simulink model "Concentrationlambdasum"  (R2020a)
settings: Solver=VariableStepAuto  StartTime=0.0  StopTime=10.0  RelTol=1e-3
undefined symbols (not defined in the file): beta1, beta2, beta3, beta4, beta5, beta6, lambda1, lambda2, lambda3, lambda4, lambda5, lambda6, mean_prompt_neutron_gen_t
settings Model: Creator=marce  LastModifiedBy=tkdmc

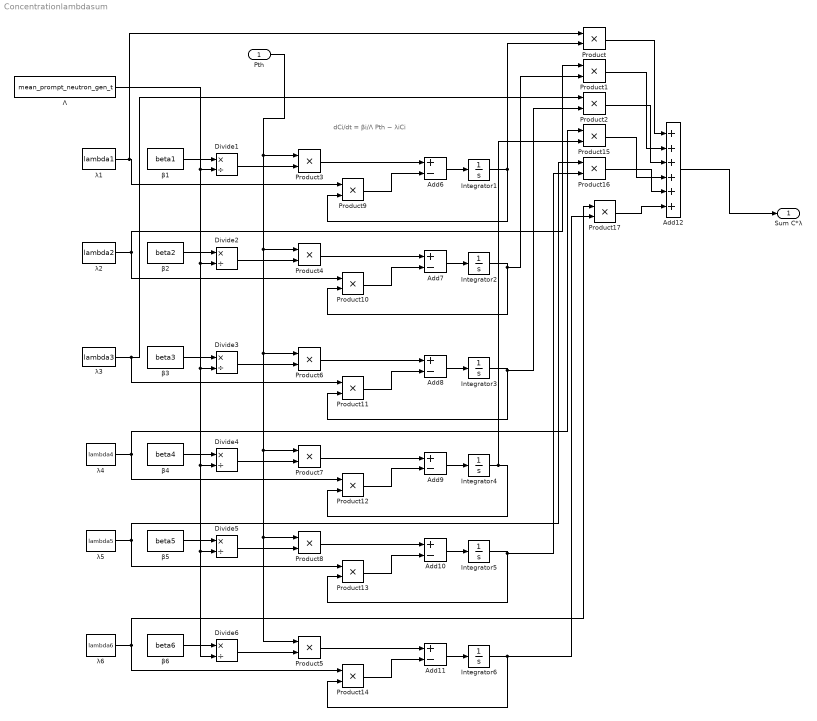
== system Concentrationlambdasum ==
  note: dCi/dt = βi/Λ Pth − λiCi
  Pth : Inport
  Add{6..11} (6 alike) : Sum  Inputs=+-
  Add12 : Sum  Inputs=++++++
  Divide{1..6} (6 alike) : Product  Inputs=*/
  Integrator{1..6} (6 alike) : Integrator
  Product{,1..17} (18 alike) : Product
  "Λ " : Constant  Value=mean_prompt_neutron_gen_t
  β1 : Constant  Value=beta1
  β2 : Constant  Value=beta2
  β3 : Constant  Value=beta3
  β4 : Constant  Value=beta4
  β5 : Constant  Value=beta5
  β6 : Constant  Value=beta6
  λ1 : Constant  Value=lambda1
  λ2 : Constant  Value=lambda2
  λ3 : Constant  Value=lambda3
  λ4 : Constant  Value=lambda4
  λ5 : Constant  Value=lambda5
  λ6 : Constant  Value=lambda6
  Sum C*λ : Outport
  wires:
  Add12/1 -> Sum C*λ/1
  Divide1/1 -> Product3/2
  β1/1 -> Divide1/1
  Product9/1 -> Add6/2
  λ6/1 -> Product14/1, Product17/1
  Product11/1 -> Add8/2
  β6/1 -> Divide6/1
  Integrator3/1 -> Product2/2, Product11/2
  Product8/1 -> Add10/1
  λ5/1 -> Product16/1, Product13/1
  Add7/1 -> Integrator2/1
  Add9/1 -> Integrator4/1
  Integrator6/1 -> Product17/2, Product14/2
  Product6/1 -> Add8/1
  Integrator2/1 -> Product1/2, Product10/2
  Divide6/1 -> Product5/2
  λ1/1 -> Product/1, Product9/1
  Product10/1 -> Add7/2
  Product3/1 -> Add6/1
  Integrator5/1 -> Product16/2, Product13/2
  λ2/1 -> Product10/1, Product1/1
  Product4/1 -> Add7/1
  β4/1 -> Divide4/1
  Add10/1 -> Integrator5/1
  β3/1 -> Divide3/1
  Divide3/1 -> Product6/2
  Divide2/1 -> Product4/2
  λ4/1 -> Product15/1, Product12/1
  Add6/1 -> Integrator1/1
  β2/1 -> Divide2/1
  Product5/1 -> Add11/1
  Divide4/1 -> Product7/2
  Integrator1/1 -> Product/2, Product9/2
  Add8/1 -> Integrator3/1
  β5/1 -> Divide5/1
  Product14/1 -> Add11/2
  Divide5/1 -> Product8/2
  Product13/1 -> Add10/2
  Pth/1 -> Product5/1, Product8/1, Product7/1, Product6/1, Product4/1, Product3/1
  Product7/1 -> Add9/1
  λ3/1 -> Product2/1, Product11/1
  Add11/1 -> Integrator6/1
  Product12/1 -> Add9/2
  Integrator4/1 -> Product12/2, Product15/2
  "Λ "/1 -> Divide6/2, Divide5/2, Divide4/2, Divide3/2, Divide2/2, Divide1/2
  Product17/1 -> Add12/6
  Product16/1 -> Add12/5
  Product15/1 -> Add12/4
  Product2/1 -> Add12/3
  Product1/1 -> Add12/2
  Product/1 -> Add12/1
